simulink library "GFL_Lib"  (R2021a)
settings: Solver=VariableStepAuto  StartTime=0.0  StopTime=10.0  RelTol=1e-3
values from neighbouring files (symbols this model uses):
  Ki_i = Rc_eq*wn_i    [Init_GFL.m]
  Kp_i = Lc_eq/wb*wn_i    [Init_GFL.m]
  Lc_eq = Lc_pu + dLc_pu    [Init_VI_mmc.m]
  Lc_pu = Lt_pu+Larm_pu/2    [Init_VI_mmc.m]
  Lf_pu = Lc_eq    [Init_GFL.m]
  Va0 = sqrt(2)*Vb1*Vvsc0*sin(Theta_vsc0*pi/180)    [Init_LF_LCL_old.m]
  Vb0 = sqrt(2)*Vb1*Vvsc0*sin(Theta_vsc0*pi/180-2*pi/3)    [Init_LF_LCL_old.m]
  Vc0 = sqrt(2)*Vb1*Vvsc0*sin(Theta_vsc0*pi/180+2*pi/3)    [Init_LF_LCL_old.m]
  Vm0_d = Vvsc0 * cos(Theta_vsc0*pi/180-Theta_m0*pi/180)    [Init_LF_LCL_old.m]
  Vm0_q = Vvsc0 * sin(Theta_vsc0*pi/180-Theta_m0*pi/180)    [Init_LF_LCL_old.m]
  Vvsc0 = abs(Vm)    [Init_LF_LCL_old.m]
undefined symbols (not defined in the file or in its folder): Carm, Diff_CC_ki, Diff_CC_kp, fb, Ib2, Idcb, Ki_Wdiff_pu, Ki_Wtot_pu, Kp_Rvi_pu, Kp_Wdiff_pu, Kp_Wtot_pu, Lb, Sb, Solver_Time_Step, Time_Step, Vb1, Vb2, Vdcb, Vm0, VSC01_id0, wb, Zb
libraries: Control_Lib x57, spsVoltageMeasurementLib x17, spsSeriesRLCBranchLib x14, spsThreePhaseSourceLib x12, spsThreePhaseBreakerLib x10, spsThreePhaseVIMeasurementLib x9, spsThreePhaseTransformerTwoWindingsLib x7, spsCurrentMeasurementLib x7, powerlib x7, spsControlledCurrentSourceLib x6, spsControlledVoltageSourceLib x6, slpidlib x6
(part 4 of 6)

== system GFL_Lib/Mean Model 2-Level L-filter_sav/Mean_Model ==
  Uref : Inport
  Constant : Constant
  Memory : Memory
  NOT1 : Logic  Operator=NOT  IconShape=distinctive  AllPortsSameDT=off  OutDataTypeStr=boolean
  Terminator : Terminator
  Three-Phase Breaker1 : spsThreePhaseBreakerLib/Three-Phase Breaker  InitialState=closed  SwitchA=on  SwitchB=on  SwitchC=on  SwitchTimes="[4/60  10/60]"  External=on  BreakerResistance=0.001  SnubberResistance=1e6  SnubberCapacitance=inf  Measurements=None
  Three-Phase Breaker2 : spsThreePhaseBreakerLib/Three-Phase Breaker  InitialState=open  SwitchA=on  SwitchB=on  SwitchC=on  SwitchTimes="[4/60  10/60]"  External=on  BreakerResistance=0.001  SnubberResistance=1e6  SnubberCapacitance=inf  Measurements=None
  Three-Phase Source : spsThreePhaseSourceLib/Three-Phase Source  InternalConnection=Yg  VoltagePhases=off  Voltage=Vvsc0*Un1  PhaseAngle=Theta_vsc0  Voltage_phases=[25e3 25e3 25e3]/sqrt(3)  PhaseAngles_phases=[0 -120 +120]  Frequency=fb  NonIdealSource=off  SpecifyImpedance=off  Resistance=0  Inductance=0  ShortCircuitLevel=100e6  BaseVoltage=VSC01_Un1  XRratio=7  BusType=swing  Pref=0.3  Qref=0  Prefabc=[10e3, 10e3, 10e3]  Qrefabc=[0, 0, 0]  Qmin=-Inf  Qmax=Inf
  Universal Bridge : spsUniversalBridgeLib/Universal Bridge  Arms=3  SnubberResistance=1e5  SnubberCapacitance=inf  Device=Average-model based VSC  Ron=1e-3  Lon=0  ForwardVoltages="[  0  0  ]"  ForwardVoltage=0  GTOparameters=[ 10e-6 , 20e-6 ]  IGBTparameters=[ 1e-6 , 2e-6 ]  Measurements=None  Measurements_2=None  converterType=Rectifier
  Vdc : spsVoltageMeasurementLib/Voltage Measurement  PhasorSimulation=off  OutputType=Complex  PSBequivalent=0
  mp3 : Gain  Gain=2/Udcn
  PhA : PMIOPort  Side=Right
  PhB : PMIOPort  Port=2  Side=Right
  PhC : PMIOPort  Port=3  Side=Right
  Vdc+ : PMIOPort  Port=4  Side=Left
  Vdc- : PMIOPort  Port=5  Side=Left
  wires:
  NOT1/1 -> Three-Phase Breaker1/1
  Memory/1 -> NOT1/1, Three-Phase Breaker2/1
  mp3/1 -> Universal Bridge/1
  Uref/1 -> mp3/1
  Vdc/1 -> Terminator/1
  Constant/1 -> Memory/1
  connections:
  Three-Phase Breaker2/LConn1 -- Three-Phase Breaker1/LConn1 -- PhA/RConn1
  Three-Phase Breaker2/LConn2 -- Three-Phase Breaker1/LConn2 -- PhB/RConn1
  Three-Phase Breaker2/LConn3 -- Three-Phase Breaker1/LConn3 -- PhC/RConn1
  Three-Phase Breaker2/RConn1 -- Universal Bridge/LConn1
  Three-Phase Breaker2/RConn2 -- Universal Bridge/LConn2
  Three-Phase Breaker2/RConn3 -- Universal Bridge/LConn3
  Three-Phase Source/RConn1 -- Three-Phase Breaker1/RConn1
  Three-Phase Source/RConn2 -- Three-Phase Breaker1/RConn2
  Three-Phase Source/RConn3 -- Three-Phase Breaker1/RConn3
  Vdc/LConn1 -- Universal Bridge/RConn1 -- Vdc+/RConn1
  Vdc/LConn2 -- Universal Bridge/RConn2 -- Vdc-/RConn1

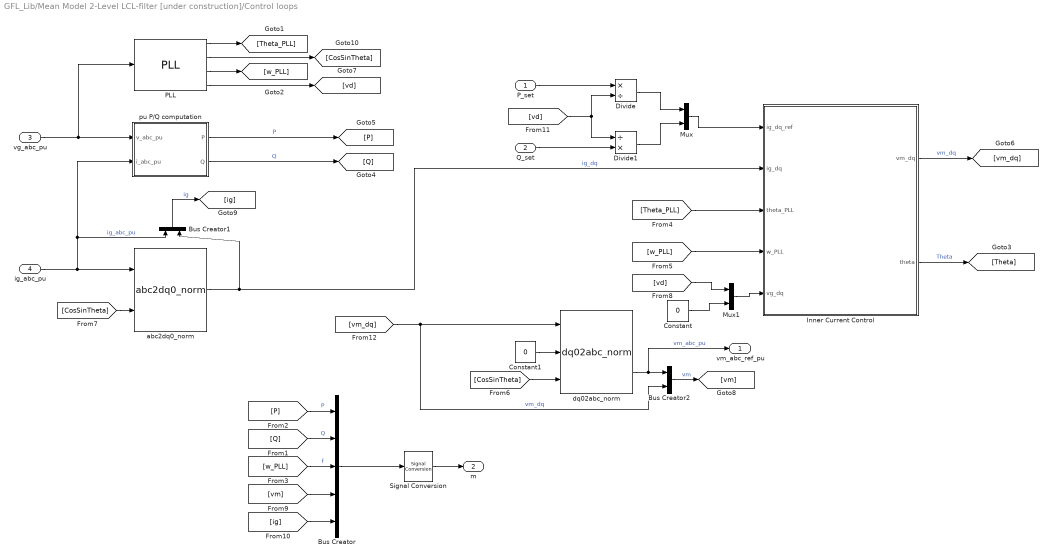
== system GFL_Lib/Mean Model 2-Level LCL-filter [under construction]/Control loops ==
  P_set : Inport
  Q_set : Inport  Port=2
  vg_abc_pu : Inport  Port=3
  ig_abc_pu : Inport  Port=4
  " pu P/Q computation" : Subsystem  DialogController=POWERSYS.PowerSysDialog
  Bus Creator : BusCreator  Inputs=5
  Bus Creator1 : BusCreator  Inputs=2
  Bus Creator2 : BusCreator  Inputs=2
  Constant : Constant  Value=0
  Constant1 : Constant  Value=0
  Divide : Product  Inputs=*/
  Divide1 : Product  Inputs=/*
  Inner Current Control : Subsystem
  Mux : Mux  Inputs=2
  Mux1 : Mux  Inputs=2
  PLL : Control_Lib/PLL  fb=fb  Tr_PLL=Tr_PLL*1000  Theta0=Theta0
      settings: SourceProductName=VSC4SPS
  Signal Conversion : SignalConversion  OverrideOpt=off
  abc2dq0_norm : Control_Lib/abc2dq0_norm  referenceAxisMode=Reference axis at 90 degrees behind phase_a  baseUpdateGain=1/sqrt(3)
      settings: SourceProductName=VSC4SPS
  dq02abc_norm : Control_Lib/dq02abc_norm  referenceAxisMode=Reference axis at 90 degrees behind phase_a  baseUpdateGain=sqrt(3)
      settings: SourceProductName=VSC4SPS
  vm_abc_ref_pu : Outport  VectorParamsAs1DForOutWhenUnconnected=off
  m : Outport  Port=2  VectorParamsAs1DForOutWhenUnconnected=off
  wires:
  PLL/3 -> [w_PLL]
  PLL/1 -> [Theta_PLL]
  [ig] -> Bus Creator/5
  Bus Creator1/1 -> [ig]  "ig"
  Bus Creator/1 -> Signal Conversion/1
  [vm] -> Bus Creator/4
  Bus Creator2/1 -> [vm]  "vm"
  [CosSinTheta] -> abc2dq0_norm/2
  [CosSinTheta] -> dq02abc_norm/3
  Inner Current Control/2(theta) -> [Theta]  "Theta"
  abc2dq0_norm/2 -> Bus Creator1/2, Inner Current Control/2(ig_dq)  "ig_dq"
  ig_abc_pu/1 -> " pu P/Q computation"/2(i_abc_pu), Bus Creator1/1, abc2dq0_norm/1  "ig_abc_pu"
  " pu P/Q computation"/1(P) -> [P]  "P"
  vg_abc_pu/1 -> " pu P/Q computation"/1(v_abc_pu), PLL/1
  Inner Current Control/1(vm_dq) -> [vm_dq]  "vm_dq"
  [w_PLL] -> Inner Current Control/4(w_PLL)
  P_set/1 -> Divide/1
  [Theta_PLL] -> Inner Current Control/3(theta_PLL)
  [vm_dq] -> dq02abc_norm/1, Bus Creator2/2  "vm_dq"
  " pu P/Q computation"/2(Q) -> [Q]  "Q"
  Q_set/1 -> Divide1/2
  dq02abc_norm/2 -> vm_abc_ref_pu/1, Bus Creator2/1  "vm_abc_pu"
  [w_PLL] -> Bus Creator/3  "f"
  [Q] -> Bus Creator/2  "Q"
  [P] -> Bus Creator/1  "P"
  Signal Conversion/1 -> m/1
  PLL/4 -> [vd]
  [vd] -> Divide/2, Divide1/1
  Divide/1 -> Mux/1
  Divide1/1 -> Mux/2
  Mux/1 -> Inner Current Control/1(ig_dq_ref)
  [vd] -> Mux1/1
  Mux1/1 -> Inner Current Control/5(vg_dq)
  Constant/1 -> Mux1/2
  PLL/2 -> [CosSinTheta]
  Constant1/1 -> dq02abc_norm/2

== system GFL_Lib/Mean Model 2-Level LCL-filter [under construction]/Mean_model ==
  Uref : Inport
  Constant : Constant
  Memory : Memory
  NOT1 : Logic  Operator=NOT  IconShape=distinctive  AllPortsSameDT=off  OutDataTypeStr=boolean
  Terminator : Terminator
  Three-Phase Breaker1 : powerlib/Elements/Three-Phase Breaker  InitialState=closed  SwitchA=on  SwitchB=on  SwitchC=on  SwitchTimes="[4/60  10/60]"  External=on  BreakerResistance=0.001  SnubberResistance=1e6  SnubberCapacitance=inf  Measurements=None
  Three-Phase Breaker2 : powerlib/Elements/Three-Phase Breaker  InitialState=open  SwitchA=on  SwitchB=on  SwitchC=on  SwitchTimes="[4/60  10/60]"  External=on  BreakerResistance=0.001  SnubberResistance=1e6  SnubberCapacitance=inf  Measurements=None
  Three-Phase Source : powerlib/Electrical Sources/Three-Phase Source  InternalConnection=Yg  VoltagePhases=off  Voltage=Vvsc0*Un1  PhaseAngle=Theta_vsc0  Voltage_phases=[25e3 25e3 25e3]/sqrt(3)  PhaseAngles_phases=[0 -120 +120]  Frequency=fb  NonIdealSource=off  SpecifyImpedance=off  Resistance=0  Inductance=0  ShortCircuitLevel=100e6  BaseVoltage=VSC01_Un1  XRratio=7  BusType=swing  Pref=0.3  Qref=0  Prefabc=[10e3, 10e3, 10e3]  Qrefabc=[0, 0, 0]  Qmin=-Inf  Qmax=Inf
  Universal Bridge : powerlib/Power Electronics/Universal Bridge  Arms=3  SnubberResistance=1e5  SnubberCapacitance=inf  Device=Average-model based VSC  Ron=1e-3  Lon=0  ForwardVoltages="[  0  0  ]"  ForwardVoltage=0  GTOparameters=[ 10e-6 , 20e-6 ]  IGBTparameters=[ 1e-6 , 2e-6 ]  Measurements=None  Measurements_2=None  converterType=Rectifier
  Vdc : powerlib/Measurements/Voltage Measurement  PhasorSimulation=off  OutputType=Complex  PSBequivalent=0
  mp3 : Gain  Gain=2/Udcn
  PhA : PMIOPort  Side=Right
  PhB : PMIOPort  Port=2  Side=Right
  PhC : PMIOPort  Port=3  Side=Right
  Vdc+ : PMIOPort  Port=4  Side=Left
  Vdc- : PMIOPort  Port=5  Side=Left
  wires:
  NOT1/1 -> Three-Phase Breaker1/1
  Memory/1 -> NOT1/1, Three-Phase Breaker2/1
  mp3/1 -> Universal Bridge/1
  Uref/1 -> mp3/1
  Vdc/1 -> Terminator/1
  Constant/1 -> Memory/1
  connections:
  Three-Phase Breaker2/LConn1 -- Three-Phase Breaker1/LConn1 -- PhA/RConn1
  Three-Phase Breaker2/LConn2 -- Three-Phase Breaker1/LConn2 -- PhB/RConn1
  Three-Phase Breaker2/LConn3 -- Three-Phase Breaker1/LConn3 -- PhC/RConn1
  Three-Phase Breaker2/RConn1 -- Universal Bridge/LConn1
  Three-Phase Breaker2/RConn2 -- Universal Bridge/LConn2
  Three-Phase Breaker2/RConn3 -- Universal Bridge/LConn3
  Three-Phase Source/RConn1 -- Three-Phase Breaker1/RConn1
  Three-Phase Source/RConn2 -- Three-Phase Breaker1/RConn2
  Three-Phase Source/RConn3 -- Three-Phase Breaker1/RConn3
  Vdc/LConn1 -- Universal Bridge/RConn1 -- Vdc+/RConn1
  Vdc/LConn2 -- Universal Bridge/RConn2 -- Vdc-/RConn1

== system GFL_Lib/GFL IDEAL VSC/Control loops/ pu P//Q computation ==
  v_abc_pu : Inport  PortDimensions=3
  i_abc_pu : Inport  Port=2  PortDimensions=3
  Demux : Demux  Outputs=3
      settings: DisplayOption=none
  Mux : Mux  Inputs=3
  Product1 : Product  InputSameDT=on  SaturateOnIntegerOverflow=on  OutDataTypeStr=Inherit: Same as first input
  Product3 : Product  InputSameDT=on  SaturateOnIntegerOverflow=on  OutDataTypeStr=Inherit: Same as first input
  Sum : Sum  Inputs=+-  InputSameDT=on  SaturateOnIntegerOverflow=on  OutDataTypeStr=Inherit: Same as first input
  Sum1 : Sum  Inputs=1  InputSameDT=on  SaturateOnIntegerOverflow=on  OutDataTypeStr=Inherit: Same as first input
  Sum4 : Sum  Inputs=1  InputSameDT=on  SaturateOnIntegerOverflow=on  OutDataTypeStr=Inherit: Same as first input
  Sum5 : Sum  Inputs=+-  InputSameDT=on  SaturateOnIntegerOverflow=on  OutDataTypeStr=Inherit: Same as first input
  Sum6 : Sum  Inputs=+-  InputSameDT=on  SaturateOnIntegerOverflow=on  OutDataTypeStr=Inherit: Same as first input
  pu->V : Gain  Gain=1/sqrt(3)  SaturateOnIntegerOverflow=on  OutDataTypeStr=Inherit: Same as input  ParamDataTypeStr=Inherit: Same as input
  pu->V1 : Gain  Gain=1/3  SaturateOnIntegerOverflow=on  OutDataTypeStr=Inherit: Same as input  ParamDataTypeStr=Inherit: Same as input
  pu->V2 : Gain  Gain=1/3  SaturateOnIntegerOverflow=on  OutDataTypeStr=Inherit: Same as input  ParamDataTypeStr=Inherit: Same as input
  P : Outport  VectorParamsAs1DForOutWhenUnconnected=off
  Q : Outport  Port=2  VectorParamsAs1DForOutWhenUnconnected=off
  wires:
  pu->V2/1 -> Q/1
  pu->V1/1 -> P/1
  Sum1/1 -> pu->V/1
  Product3/1 -> Sum1/1
  Product1/1 -> Sum4/1
  v_abc_pu/1 -> Product1/1, Demux/1
  i_abc_pu/1 -> Product1/2, Product3/2
  Sum4/1 -> pu->V1/1
  Demux/1 -> Sum/1, Sum6/2
  Demux/2 -> Sum/2, Sum5/1
  Demux/3 -> Sum5/2, Sum6/1
  Sum/1 -> Mux/3
  Sum5/1 -> Mux/1
  Sum6/1 -> Mux/2
  Mux/1 -> Product3/1
  pu->V/1 -> pu->V2/1  "Q"

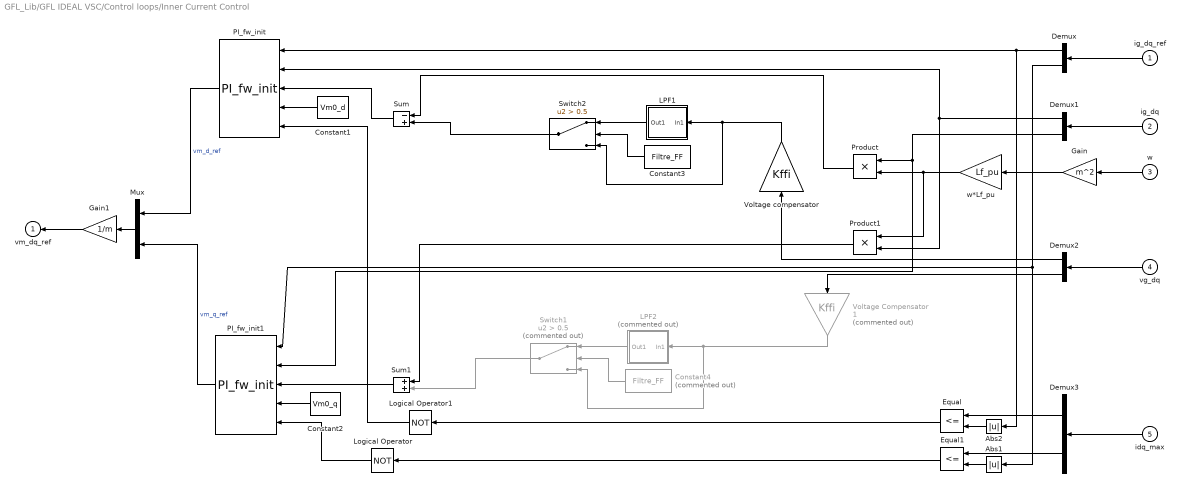
== system GFL_Lib/GFL IDEAL VSC/Control loops/Inner Current Control ==
  ig_dq_ref : Inport
  ig_dq : Inport  Port=2
  w : Inport  Port=3
  vg_dq : Inport  Port=4
  idq_max : Inport  Port=5
  Abs1 : Abs
  Abs2 : Abs
  Constant1 : Constant  Value=Vm0_d
  Constant2 : Constant  Value=Vm0_q
  Constant3 : Constant  Value=Filtre_FF
  Constant4 : Constant  Commented=on  Value=Filtre_FF
  Demux{,1..3} (4 alike) : Demux  Outputs=2
  Equal : RelationalOperator  Operator=<=  OutDataTypeStr=boolean  RndMeth=Simplest
  Equal1 : RelationalOperator  Operator=<=  OutDataTypeStr=boolean  RndMeth=Simplest
  Gain : Gain  Gain=m^2
  Gain1 : Gain  Gain=1/m
  LPF1 : Subsystem
  LPF2 : Subsystem  Commented=on
  Logical Operator : Logic  Operator=NOT  AllPortsSameDT=off  OutDataTypeStr=boolean
  Logical Operator1 : Logic  Operator=NOT  AllPortsSameDT=off  OutDataTypeStr=boolean
  Mux : Mux  Inputs=[1 1]
  PI_fw_init : Control_Lib/PI_fw_init  Kp=Kp_i  Ki=Ki_i
      settings: SourceProductName=VSC4SPS
  PI_fw_init1 : Control_Lib/PI_fw_init  Kp=Kp_i  Ki=Ki_i
      settings: SourceProductName=VSC4SPS
  Product : Product  RndMeth=Zero
  Product1 : Product  RndMeth=Zero
  Sum : Sum  Inputs=-+
  Sum1 : Sum
  Switch1 : Switch  Commented=on  Criteria=u2 > Threshold  Threshold=0.5
  Switch2 : Switch  Criteria=u2 > Threshold  Threshold=0.5
  Voltage Compensator 1 : Gain  Commented=on  Gain=Kffi
  Voltage compensator : Gain  Gain=Kffi
  w*Lf_pu : Gain  Gain=Lf_pu
  vm_dq_ref : Outport  InitialOutput=0  VectorParamsAs1DForOutWhenUnconnected=off
  wires:
  Switch1/1 -> Sum1/2
  Constant4/1 -> Switch1/2
  Voltage Compensator 1/1 -> LPF2/1(In1), Switch1/3
  LPF2/1(Out1) -> Switch1/1
  Constant3/1 -> Switch2/2
  LPF1/1(Out1) -> Switch2/1
  Gain1/1 -> vm_dq_ref/1
  Gain/1 -> w*Lf_pu/1
  Equal1/1 -> Logical Operator/1
  Equal/1 -> Logical Operator1/1
  Abs1/1 -> Equal1/2
  Abs2/1 -> Equal/2
  Demux3/2 -> Equal1/1
  Demux3/1 -> Equal/1
  idq_max/1 -> Demux3/1
  Demux2/2 -> Voltage Compensator 1/1
  Demux2/1 -> Voltage compensator/1
  Constant2/1 -> PI_fw_init1/4
  Constant1/1 -> PI_fw_init/4
  Product/1 -> Sum/1
  vg_dq/1 -> Demux2/1
  ig_dq/1 -> Demux1/1
  ig_dq_ref/1 -> Demux/1
  Demux/1 -> Abs2/1, PI_fw_init/1
  Demux1/1 -> Product1/2, PI_fw_init/2
  w*Lf_pu/1 -> Product1/1, Product/2
  Demux1/2 -> Product/1, PI_fw_init1/2
  Mux/1 -> Gain1/1
  Demux/2 -> PI_fw_init1/1, Abs1/1
  Product1/1 -> Sum1/1
  PI_fw_init/1 -> Mux/1  "vm_d_ref"
  PI_fw_init1/1 -> Mux/2  "vm_q_ref"
  w/1 -> Gain/1
  Voltage compensator/1 -> LPF1/1(In1), Switch2/3
  Sum/1 -> PI_fw_init/3
  Sum1/1 -> PI_fw_init1/3
  Switch2/1 -> Sum/2
  Logical Operator/1 -> PI_fw_init1/5
  Logical Operator1/1 -> PI_fw_init/5

== system GFL_Lib/GFL IDEAL VSC/Control loops/LPF ==
  In1 : Inport
  Add : Sum  Inputs=+-
  Gain : Gain  Gain=w_LPF
  Integrator : Integrator  InitialConditionSource=external  InitialCondition=P0
  Out1 : Outport
  wires:
  Add/1 -> Gain/1
  Gain/1 -> Integrator/1
  Integrator/1 -> Out1/1, Add/2
  In1/1 -> Integrator/2, Add/1

== system GFL_Lib/GFL IDEAL VSC/Control loops/LPF1 ==
  In1 : Inport
  Add : Sum  Inputs=+-
  Gain : Gain  Gain=w_LPF
  Integrator : Integrator  InitialConditionSource=external  InitialCondition=V0
  Ref : Outport
  wires:
  Add/1 -> Gain/1
  Gain/1 -> Integrator/1
  Integrator/1 -> Ref/1, Add/2
  In1/1 -> Integrator/2, Add/1

== system GFL_Lib/GFL IDEAL VSC/Control loops/LPF2 ==
  In1 : Inport
  Add : Sum  Inputs=+-
  Gain : Gain  Gain=w_LPF
  Integrator : Integrator  InitialConditionSource=external  InitialCondition=Q0
  Out1 : Outport
  wires:
  Add/1 -> Gain/1
  Gain/1 -> Integrator/1
  Integrator/1 -> Out1/1, Add/2
  In1/1 -> Integrator/2, Add/1

== system GFL_Lib/GFL IDEAL VSC/Control loops/LPF3 ==
  In1 : Inport
  Add : Sum  Inputs=+-
  Gain : Gain  Gain=2*pi*50
  Integrator : Integrator  InitialConditionSource=external  InitialCondition=V0
  Out1 : Outport
  wires:
  Add/1 -> Gain/1
  Gain/1 -> Integrator/1
  Integrator/1 -> Out1/1, Add/2
  In1/1 -> Integrator/2, Add/1

== system GFL_Lib/GFL IDEAL VSC/Control loops/RMS derivation ==
  dq : Inport
  Demux : Demux  Outputs=2
  Sqrt : Sqrt  SaturateOnIntegerOverflow=on
  Square : Math  Operator=square  SaturateOnIntegerOverflow=on
  Square1 : Math  Operator=square  SaturateOnIntegerOverflow=on
  Sum : Sum
  rms : Outport
  wires:
  Square1/1 -> Sum/2
  Sum/1 -> Sqrt/1
  Sqrt/1 -> rms/1
  Demux/1 -> Square/1
  Square/1 -> Sum/1
  Demux/2 -> Square1/1
  dq/1 -> Demux/1

== system GFL_Lib/GFL IDEAL VSC/Control loops/RMS derivation1 ==
  dq : Inport
  Demux : Demux  Outputs=2
  Sqrt : Sqrt  SaturateOnIntegerOverflow=on
  Square : Math  Operator=square  SaturateOnIntegerOverflow=on
  Square1 : Math  Operator=square  SaturateOnIntegerOverflow=on
  Sum : Sum
  rms : Outport
  wires:
  dq/1 -> Demux/1
  Demux/2 -> Square1/1
  Square/1 -> Sum/1
  Demux/1 -> Square/1
  Sqrt/1 -> rms/1
  Sum/1 -> Sqrt/1
  Square1/1 -> Sum/2

== system GFL_Lib/GFL IDEAL VSC/Control loops/RMS derivation2 ==
  dq : Inport
  Demux : Demux  Outputs=2
  Sqrt : Sqrt  SaturateOnIntegerOverflow=on
  Square : Math  Operator=square  SaturateOnIntegerOverflow=on
  Square1 : Math  Operator=square  SaturateOnIntegerOverflow=on
  Sum : Sum
  rms : Outport
  wires:
  dq/1 -> Demux/1
  Demux/2 -> Square1/1
  Square/1 -> Sum/1
  Demux/1 -> Square/1
  Sqrt/1 -> rms/1
  Sum/1 -> Sqrt/1
  Square1/1 -> Sum/2

== system GFL_Lib/GFL IDEAL VSC/Control loops/norm1 ==
  In1 : Inport
  Add : Sum
  Demux : Demux  Outputs=2
  Sqrt : Sqrt  SaturateOnIntegerOverflow=on
  Square : Math  Operator=square  SaturateOnIntegerOverflow=on
  Square1 : Math  Operator=square  SaturateOnIntegerOverflow=on
  Out1 : Outport
  wires:
  Sqrt/1 -> Out1/1
  Add/1 -> Sqrt/1
  Demux/2 -> Square1/1
  Demux/1 -> Square/1
  Square/1 -> Add/1
  Square1/1 -> Add/2
  In1/1 -> Demux/1

== system GFL_Lib/GFL IDEAL VSC/Control loops/norm2 ==
  In1 : Inport
  Add : Sum
  Demux : Demux  Outputs=2
  Sqrt : Sqrt  SaturateOnIntegerOverflow=on
  Square : Math  Operator=square  SaturateOnIntegerOverflow=on
  Square1 : Math  Operator=square  SaturateOnIntegerOverflow=on
  Out1 : Outport
  wires:
  Sqrt/1 -> Out1/1
  Add/1 -> Sqrt/1
  Demux/2 -> Square1/1
  Demux/1 -> Square/1
  Square/1 -> Add/1
  Square1/1 -> Add/2
  In1/1 -> Demux/1

== system GFL_Lib/GFL MMC/Control loops/ pu P//Q computation ==
  v_abc_pu : Inport  PortDimensions=3
  i_abc_pu : Inport  Port=2  PortDimensions=3
  Demux : Demux  Outputs=3
      settings: DisplayOption=none
  Mux : Mux  Inputs=3
  Product1 : Product  InputSameDT=on  SaturateOnIntegerOverflow=on  OutDataTypeStr=Inherit: Same as first input
  Product3 : Product  InputSameDT=on  SaturateOnIntegerOverflow=on  OutDataTypeStr=Inherit: Same as first input
  Sum : Sum  Inputs=+-  InputSameDT=on  SaturateOnIntegerOverflow=on  OutDataTypeStr=Inherit: Same as first input
  Sum1 : Sum  Inputs=1  InputSameDT=on  SaturateOnIntegerOverflow=on  OutDataTypeStr=Inherit: Same as first input
  Sum4 : Sum  Inputs=1  InputSameDT=on  SaturateOnIntegerOverflow=on  OutDataTypeStr=Inherit: Same as first input
  Sum5 : Sum  Inputs=+-  InputSameDT=on  SaturateOnIntegerOverflow=on  OutDataTypeStr=Inherit: Same as first input
  Sum6 : Sum  Inputs=+-  InputSameDT=on  SaturateOnIntegerOverflow=on  OutDataTypeStr=Inherit: Same as first input
  pu->V : Gain  Gain=1/sqrt(3)  SaturateOnIntegerOverflow=on  OutDataTypeStr=Inherit: Same as input  ParamDataTypeStr=Inherit: Same as input
  pu->V1 : Gain  Gain=1/3  SaturateOnIntegerOverflow=on  OutDataTypeStr=Inherit: Same as input  ParamDataTypeStr=Inherit: Same as input
  pu->V2 : Gain  Gain=1/3  SaturateOnIntegerOverflow=on  OutDataTypeStr=Inherit: Same as input  ParamDataTypeStr=Inherit: Same as input
  P : Outport  VectorParamsAs1DForOutWhenUnconnected=off
  Q : Outport  Port=2  VectorParamsAs1DForOutWhenUnconnected=off
  wires:
  pu->V2/1 -> Q/1
  pu->V1/1 -> P/1
  Sum1/1 -> pu->V/1
  Product3/1 -> Sum1/1
  Product1/1 -> Sum4/1
  v_abc_pu/1 -> Product1/1, Demux/1
  i_abc_pu/1 -> Product1/2, Product3/2
  Sum4/1 -> pu->V1/1
  Demux/1 -> Sum/1, Sum6/2
  Demux/2 -> Sum/2, Sum5/1
  Demux/3 -> Sum5/2, Sum6/1
  Sum/1 -> Mux/3
  Sum5/1 -> Mux/1
  Sum6/1 -> Mux/2
  Mux/1 -> Product3/1
  pu->V/1 -> pu->V2/1  "Q"

== system GFL_Lib/GFL MMC/Control loops/Inner Current Control ==
  ig_dq_ref : Inport
  ig_dq : Inport  Port=2
  w : Inport  Port=3
  vg_dq : Inport  Port=4
  idq_max : Inport  Port=5
  Abs1 : Abs
  Abs2 : Abs
  Constant1 : Constant  Value=Vm0_d
  Constant2 : Constant  Value=Vm0_q
  Constant3 : Constant  Value=Filtre_FF
  Constant4 : Constant  Commented=on  Value=Filtre_FF
  Demux{,1..3} (4 alike) : Demux  Outputs=2
  Equal : RelationalOperator  Operator=<=  OutDataTypeStr=boolean  RndMeth=Simplest
  Equal1 : RelationalOperator  Operator=<=  OutDataTypeStr=boolean  RndMeth=Simplest
  Gain : Gain  Gain=m^2
  Gain1 : Gain  Gain=1/m
  LPF1 : Subsystem
  LPF2 : Subsystem  Commented=on
  Logical Operator : Logic  Operator=NOT  AllPortsSameDT=off  OutDataTypeStr=boolean
  Logical Operator1 : Logic  Operator=NOT  AllPortsSameDT=off  OutDataTypeStr=boolean
  Mux : Mux  Inputs=[1 1]
  PI_fw_init : Control_Lib/PI_fw_init  Kp=Kp_i  Ki=Ki_i
      settings: SourceProductName=VSC4SPS
  PI_fw_init1 : Control_Lib/PI_fw_init  Kp=Kp_i  Ki=Ki_i
      settings: SourceProductName=VSC4SPS
  Product : Product  RndMeth=Zero
  Product1 : Product  RndMeth=Zero
  Sum : Sum  Inputs=-+
  Sum1 : Sum
  Switch1 : Switch  Commented=on  Criteria=u2 > Threshold  Threshold=0.5
  Switch2 : Switch  Criteria=u2 > Threshold  Threshold=0.5
  Voltage Compensator 1 : Gain  Commented=on  Gain=Kffi
  Voltage compensator : Gain  Gain=Kffi
  w*Lf_pu : Gain  Gain=Lf_pu
  vm_dq_ref : Outport  InitialOutput=0  VectorParamsAs1DForOutWhenUnconnected=off
  wires:
  Switch1/1 -> Sum1/2
  Constant4/1 -> Switch1/2
  Voltage Compensator 1/1 -> LPF2/1(In1), Switch1/3
  LPF2/1(Out1) -> Switch1/1
  Constant3/1 -> Switch2/2
  LPF1/1(Out1) -> Switch2/1
  Gain1/1 -> vm_dq_ref/1
  Gain/1 -> w*Lf_pu/1
  Equal1/1 -> Logical Operator/1
  Equal/1 -> Logical Operator1/1
  Abs1/1 -> Equal1/2
  Abs2/1 -> Equal/2
  Demux3/2 -> Equal1/1
  Demux3/1 -> Equal/1
  idq_max/1 -> Demux3/1
  Demux2/2 -> Voltage Compensator 1/1
  Demux2/1 -> Voltage compensator/1
  Constant2/1 -> PI_fw_init1/4
  Constant1/1 -> PI_fw_init/4
  Product/1 -> Sum/1
  vg_dq/1 -> Demux2/1
  ig_dq/1 -> Demux1/1
  ig_dq_ref/1 -> Demux/1
  Demux/1 -> Abs2/1, PI_fw_init/1
  Demux1/1 -> Product1/2, PI_fw_init/2
  w*Lf_pu/1 -> Product1/1, Product/2
  Demux1/2 -> Product/1, PI_fw_init1/2
  Mux/1 -> Gain1/1
  Demux/2 -> PI_fw_init1/1, Abs1/1
  Product1/1 -> Sum1/1
  PI_fw_init/1 -> Mux/1  "vm_d_ref"
  PI_fw_init1/1 -> Mux/2  "vm_q_ref"
  w/1 -> Gain/1
  Voltage compensator/1 -> LPF1/1(In1), Switch2/3
  Sum/1 -> PI_fw_init/3
  Sum1/1 -> PI_fw_init1/3
  Switch2/1 -> Sum/2
  Logical Operator/1 -> PI_fw_init1/5
  Logical Operator1/1 -> PI_fw_init/5

== system GFL_Lib/GFL MMC/Control loops/LPF ==
  In1 : Inport
  Add : Sum  Inputs=+-
  Gain : Gain  Gain=w_LPF
  Integrator : Integrator  InitialConditionSource=external  InitialCondition=P0
  Out1 : Outport
  wires:
  Add/1 -> Gain/1
  Gain/1 -> Integrator/1
  Integrator/1 -> Out1/1, Add/2
  In1/1 -> Integrator/2, Add/1

== system GFL_Lib/GFL MMC/Control loops/LPF1 ==
  In1 : Inport
  Add : Sum  Inputs=+-
  Gain : Gain  Gain=w_LPF
  Integrator : Integrator  InitialConditionSource=external  InitialCondition=V0
  Out1 : Outport
  wires:
  Add/1 -> Gain/1
  Gain/1 -> Integrator/1
  Integrator/1 -> Out1/1, Add/2
  In1/1 -> Integrator/2, Add/1

== system GFL_Lib/GFL MMC/Control loops/LPF2 ==
  In1 : Inport
  Add : Sum  Inputs=+-
  Gain : Gain  Gain=w_LPF
  Integrator : Integrator  InitialConditionSource=external  InitialCondition=Q0
  Out1 : Outport
  wires:
  Add/1 -> Gain/1
  Gain/1 -> Integrator/1
  Integrator/1 -> Out1/1, Add/2
  In1/1 -> Integrator/2, Add/1

== system GFL_Lib/GFL MMC/Control loops/LPF3 ==
  In1 : Inport
  Add : Sum  Inputs=+-
  Gain : Gain  Gain=2*pi*50
  Integrator : Integrator  InitialConditionSource=external  InitialCondition=V0
  Out1 : Outport
  wires:
  Add/1 -> Gain/1
  Gain/1 -> Integrator/1
  Integrator/1 -> Out1/1, Add/2
  In1/1 -> Integrator/2, Add/1

== system GFL_Lib/GFL MMC/Control loops/RMS derivation ==
  dq : Inport
  Demux : Demux  Outputs=2
  Sqrt : Sqrt  SaturateOnIntegerOverflow=on
  Square : Math  Operator=square  SaturateOnIntegerOverflow=on
  Square1 : Math  Operator=square  SaturateOnIntegerOverflow=on
  Sum : Sum
  rms : Outport
  wires:
  Square1/1 -> Sum/2
  Sum/1 -> Sqrt/1
  Sqrt/1 -> rms/1
  Demux/1 -> Square/1
  Square/1 -> Sum/1
  Demux/2 -> Square1/1
  dq/1 -> Demux/1

== system GFL_Lib/GFL MMC/Control loops/RMS derivation1 ==
  dq : Inport
  Demux : Demux  Outputs=2
  Sqrt : Sqrt  SaturateOnIntegerOverflow=on
  Square : Math  Operator=square  SaturateOnIntegerOverflow=on
  Square1 : Math  Operator=square  SaturateOnIntegerOverflow=on
  Sum : Sum
  rms : Outport
  wires:
  dq/1 -> Demux/1
  Demux/2 -> Square1/1
  Square/1 -> Sum/1
  Demux/1 -> Square/1
  Sqrt/1 -> rms/1
  Sum/1 -> Sqrt/1
  Square1/1 -> Sum/2

== system GFL_Lib/GFL MMC/Control loops/RMS derivation2 ==
  dq : Inport
  Demux : Demux  Outputs=2
  Sqrt : Sqrt  SaturateOnIntegerOverflow=on
  Square : Math  Operator=square  SaturateOnIntegerOverflow=on
  Square1 : Math  Operator=square  SaturateOnIntegerOverflow=on
  Sum : Sum
  rms : Outport
  wires:
  dq/1 -> Demux/1
  Demux/2 -> Square1/1
  Square/1 -> Sum/1
  Demux/1 -> Square/1
  Sqrt/1 -> rms/1
  Sum/1 -> Sqrt/1
  Square1/1 -> Sum/2

== system GFL_Lib/GFL MMC/Control loops/norm1 ==
  In1 : Inport
  Add : Sum
  Demux : Demux  Outputs=2
  Sqrt : Sqrt  SaturateOnIntegerOverflow=on
  Square : Math  Operator=square  SaturateOnIntegerOverflow=on
  Square1 : Math  Operator=square  SaturateOnIntegerOverflow=on
  Out1 : Outport
  wires:
  Sqrt/1 -> Out1/1
  Add/1 -> Sqrt/1
  Demux/2 -> Square1/1
  Demux/1 -> Square/1
  Square/1 -> Add/1
  Square1/1 -> Add/2
  In1/1 -> Demux/1

== system GFL_Lib/GFL MMC/Control loops/norm2 ==
  In1 : Inport
  Add : Sum
  Demux : Demux  Outputs=2
  Sqrt : Sqrt  SaturateOnIntegerOverflow=on
  Square : Math  Operator=square  SaturateOnIntegerOverflow=on
  Square1 : Math  Operator=square  SaturateOnIntegerOverflow=on
  Out1 : Outport
  wires:
  Sqrt/1 -> Out1/1
  Add/1 -> Sqrt/1
  Demux/2 -> Square1/1
  Demux/1 -> Square/1
  Square/1 -> Add/1
  Square1/1 -> Add/2
  In1/1 -> Demux/1

== system GFL_Lib/GFM_VC MMC/Bridge_Model/Decoupling voltage ==
  Vv_ref : Inport
  Vdiff_ref : Inport  Port=2
  Sum7 : Sum  Inputs=+-
  Sum8 : Sum
  Vmu_ref : Outport
  Vml_ref : Outport  Port=2
  wires:
  Sum8/1 -> Vml_ref/1  "Ul"
  Sum7/1 -> Vmu_ref/1
  Vdiff_ref/1 -> Sum8/1, Sum7/1
  Vv_ref/1 -> Sum8/2, Sum7/2

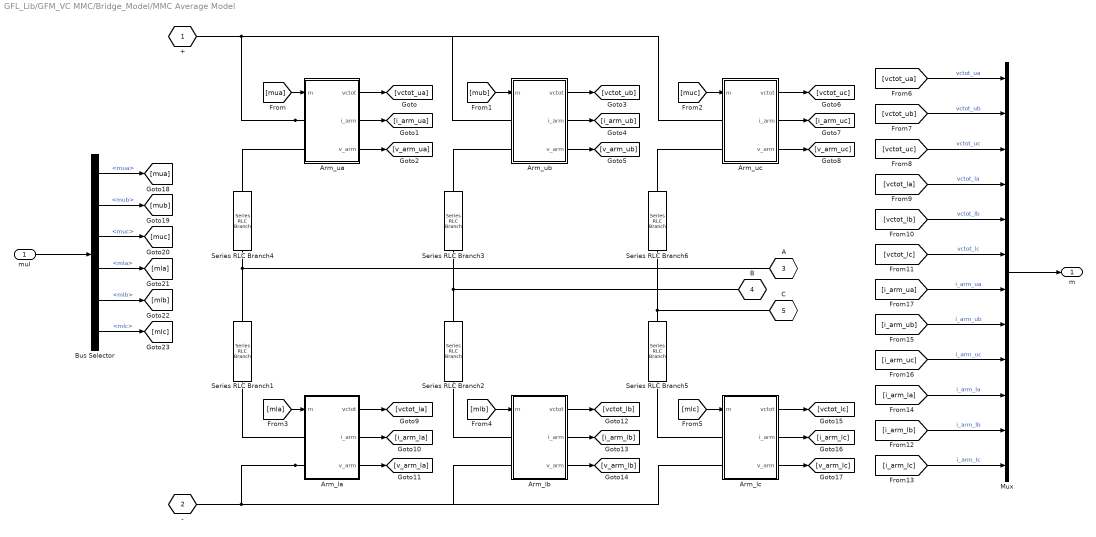
== system GFL_Lib/GFM_VC MMC/Bridge_Model/MMC Average Model ==
  mul : Inport
  Arm_la : Subsystem  mask{C_arm=Carm, Vdc=Udcn}
      mask prompts: C_arm "Arm equivalent Capacitor (F)"; Vdc "Init DC Voltage (V)"
  Arm_lb : Subsystem  mask{C_arm=Carm, Vdc=Udcn}
      mask prompts: C_arm "Arm equivalent Capacitor (F)"; Vdc "Init DC Voltage (V)"
  Arm_lc : Subsystem  mask{C_arm=Carm, Vdc=Udcn}
      mask prompts: C_arm "Arm equivalent Capacitor (F)"; Vdc "Init DC Voltage (V)"
  Arm_ua : Subsystem  mask{C_arm=Carm, Vdc=Udcn}
      mask prompts: C_arm "Arm equivalent Capacitor (F)"; Vdc "Init DC Voltage (V)"
  Arm_ub : Subsystem  mask{C_arm=Carm, Vdc=Udcn}
      mask prompts: C_arm "Arm equivalent Capacitor (F)"; Vdc "Init DC Voltage (V)"
  Arm_uc : Subsystem  mask{C_arm=Carm, Vdc=Udcn}
      mask prompts: C_arm "Arm equivalent Capacitor (F)"; Vdc "Init DC Voltage (V)"
  Bus Selector : BusSelector  OutputSignals=mua,mub,muc,mla,mlb,mlc
  Mux : Mux  Inputs=12
  Series RLC Branch{1..6} (6 alike) : spsSeriesRLCBranchLib/Series RLC Branch  LConnTagsString=__new0  RConnTagsString=__new0  BranchType=RL  Resistance=Rarm_pu*Zb  Inductance=Larm_pu*Lb  SetiL0=off  InitialCurrent=0  Capacitance=1e-6  Setx0=off  InitialVoltage=0  Measurements=None
  + : PMIOPort  Tag=PMCPort  Side=Right
  - : PMIOPort  Tag=PMCPort  Port=2  Side=Right
  A : PMIOPort  Tag=PMCPort  Port=3  Side=Left
  B : PMIOPort  Tag=PMCPort  Port=4  Side=Left
  C : PMIOPort  Tag=PMCPort  Port=5  Side=Left
  m : Outport
  wires:
  [mlb] -> Arm_lb/1(m)
  [mlc] -> Arm_lc/1(m)
  [mla] -> Arm_la/1(m)
  Arm_uc/1(vctot) -> [vctot_uc]
  Arm_lb/3(v_arm) -> [v_arm_lb]
  Arm_ub/3(v_arm) -> [v_arm_ub]
  Arm_ua/1(vctot) -> [vctot_ua]
  Arm_uc/2(i_arm) -> [i_arm_uc]
  Arm_lc/1(vctot) -> [vctot_lc]
  Arm_la/2(i_arm) -> [i_arm_la]
  Arm_la/1(vctot) -> [vctot_la]
  Arm_ub/2(i_arm) -> [i_arm_ub]
  Arm_lc/3(v_arm) -> [v_arm_lc]
  Arm_la/3(v_arm) -> [v_arm_la]
  [mua] -> Arm_ua/1(m)
  Arm_ub/1(vctot) -> [vctot_ub]
  Arm_lb/1(vctot) -> [vctot_lb]
  [mub] -> Arm_ub/1(m)
  Arm_uc/3(v_arm) -> [v_arm_uc]
  Arm_lb/2(i_arm) -> [i_arm_lb]
  Arm_ua/2(i_arm) -> [i_arm_ua]
  Arm_lc/2(i_arm) -> [i_arm_lc]
  [muc] -> Arm_uc/1(m)
  Arm_ua/3(v_arm) -> [v_arm_ua]
  mul/1 -> Bus Selector/1
  Bus Selector/1 -> [mua]  "<mua>"
  Bus Selector/2 -> [mub]  "<mub>"
  Bus Selector/3 -> [muc]  "<muc>"
  Bus Selector/6 -> [mlc]  "<mlc>"
  Bus Selector/5 -> [mlb]  "<mlb>"
  Bus Selector/4 -> [mla]  "<mla>"
  [vctot_lc] -> Mux/6  "vctot_lc"
  [vctot_uc] -> Mux/3  "vctot_uc"
  [i_arm_ua] -> Mux/7  "i_arm_ua"
  [i_arm_ub] -> Mux/8  "i_arm_ub"
  [vctot_lb] -> Mux/5  "vctot_lb"
  [i_arm_la] -> Mux/10  "i_arm_la"
  [vctot_ub] -> Mux/2  "vctot_ub"
  [i_arm_uc] -> Mux/9  "i_arm_uc"
  [vctot_la] -> Mux/4  "vctot_la"
  [i_arm_lb] -> Mux/11  "i_arm_lb"
  [vctot_ua] -> Mux/1  "vctot_ua"
  [i_arm_lc] -> Mux/12  "i_arm_lc"
  Mux/1 -> m/1
  connections:
  Series RLC Branch5/RConn1 -- Arm_lc/LConn1
  Arm_ua/LConn2 -- Series RLC Branch4/LConn1
  Series RLC Branch6/LConn1 -- Arm_uc/LConn2
  Series RLC Branch5/LConn1 -- Series RLC Branch6/RConn1 -- C/RConn1
  Series RLC Branch2/LConn1 -- B/RConn1 -- Series RLC Branch3/RConn1
  Arm_ub/LConn2 -- Series RLC Branch3/LConn1
  Series RLC Branch2/RConn1 -- Arm_lb/LConn1
  Series RLC Branch1/LConn1 -- Series RLC Branch4/RConn1 -- A/RConn1
  Arm_la/LConn2 -- -/RConn1 -- Arm_lc/LConn2 -- Arm_lb/LConn2
  Series RLC Branch1/RConn1 -- Arm_la/LConn1
  Arm_ua/LConn1 -- +/RConn1 -- Arm_uc/LConn1 -- Arm_ub/LConn1

== system GFL_Lib/GFM_VC MMC/Bridge_Model/Modulation Index Generation ==
  vmu_ref : Inport
  vml_ref : Inport  Port=2
  "1 -> Activer filtre notch 0 -> Désactiver filtre notch2" : Constant  Value=Udcn
  Bus Creator : BusCreator  Inputs=6
  Constant : Constant  Value=MMC_Control_Type
  Constant1 : Constant  Value=MMC_Control_Type
  Demux : Demux  Outputs=3
  Demux1 : Demux  Outputs=3
  Demux2 : Demux  Outputs=[3 3]
  Divide1 : Product  Inputs=/*
  Divide4 : Product  Inputs=*/
  Multiport Switch : MultiPortSwitch  Inputs=2
  Multiport Switch1 : MultiPortSwitch  Inputs=2
  Selector : Selector  InputPortWidth=12  IndexOptions=Index vector (dialog)  Indices=[1 2 3 4 5 6]  OutputSizes=1
  m limiter low : Saturate  UpperLimit=1  LowerLimit=0
  m limiter up : Saturate  UpperLimit=1  LowerLimit=0
  mul : Outport
  wires:
  Constant1/1 -> Multiport Switch1/1
  Constant/1 -> Multiport Switch/1
  Demux/3 -> Bus Creator/3  "muc"
  vmu_ref/1 -> Divide1/2
  Multiport Switch/1 -> Divide1/1
  Bus Creator/1 -> mul/1
  Demux1/1 -> Bus Creator/4  "mla"
  Demux1/2 -> Bus Creator/5  "mlb"
  Divide4/1 -> m limiter low/1
  Demux1/3 -> Bus Creator/6  "mlc"
  Multiport Switch1/1 -> Divide4/2
  Demux/2 -> Bus Creator/2  "mub"
  vml_ref/1 -> Divide4/1
  Demux/1 -> Bus Creator/1  "mua"
  m limiter up/1 -> Demux/1
  Divide1/1 -> m limiter up/1
  m limiter low/1 -> Demux1/1
  "1 -> Activer filtre notch 0 -> Désactiver filtre notch2"/1 -> Multiport Switch/2, Multiport Switch1/2
  Selector/1 -> Demux2/1
  [m_mmc] -> Selector/1
  Demux2/1 -> Multiport Switch/3
  Demux2/2 -> Multiport Switch1/3

== system GFL_Lib/GFM_VC MMC/Control loops/ pu P//Q computation ==
  v_abc_pu : Inport  PortDimensions=3
  i_abc_pu : Inport  Port=2  PortDimensions=3
  Demux : Demux  Outputs=3
      settings: DisplayOption=none
  Mux : Mux  Inputs=3
  Product1 : Product  InputSameDT=on  SaturateOnIntegerOverflow=on  OutDataTypeStr=Inherit: Same as first input
  Product3 : Product  InputSameDT=on  SaturateOnIntegerOverflow=on  OutDataTypeStr=Inherit: Same as first input
  Sum : Sum  Inputs=+-  InputSameDT=on  SaturateOnIntegerOverflow=on  OutDataTypeStr=Inherit: Same as first input
  Sum1 : Sum  Inputs=1  InputSameDT=on  SaturateOnIntegerOverflow=on  OutDataTypeStr=Inherit: Same as first input
  Sum4 : Sum  Inputs=1  InputSameDT=on  SaturateOnIntegerOverflow=on  OutDataTypeStr=Inherit: Same as first input
  Sum5 : Sum  Inputs=+-  InputSameDT=on  SaturateOnIntegerOverflow=on  OutDataTypeStr=Inherit: Same as first input
  Sum6 : Sum  Inputs=+-  InputSameDT=on  SaturateOnIntegerOverflow=on  OutDataTypeStr=Inherit: Same as first input
  pu->V : Gain  Gain=1/sqrt(3)  SaturateOnIntegerOverflow=on  OutDataTypeStr=Inherit: Same as input  ParamDataTypeStr=Inherit: Same as input
  pu->V1 : Gain  Gain=1/3  SaturateOnIntegerOverflow=on  OutDataTypeStr=Inherit: Same as input  ParamDataTypeStr=Inherit: Same as input
  pu->V2 : Gain  Gain=1/3  SaturateOnIntegerOverflow=on  OutDataTypeStr=Inherit: Same as input  ParamDataTypeStr=Inherit: Same as input
  P : Outport  VectorParamsAs1DForOutWhenUnconnected=off
  Q : Outport  Port=2  VectorParamsAs1DForOutWhenUnconnected=off
  wires:
  pu->V2/1 -> Q/1
  pu->V1/1 -> P/1
  Sum1/1 -> pu->V/1
  Product3/1 -> Sum1/1
  Product1/1 -> Sum4/1
  v_abc_pu/1 -> Product1/1, Demux/1
  i_abc_pu/1 -> Product1/2, Product3/2
  Sum4/1 -> pu->V1/1
  Demux/1 -> Sum/1, Sum6/2
  Demux/2 -> Sum/2, Sum5/1
  Demux/3 -> Sum5/2, Sum6/1
  Sum/1 -> Mux/3
  Sum5/1 -> Mux/1
  Sum6/1 -> Mux/2
  Mux/1 -> Product3/1
  pu->V/1 -> pu->V2/1  "Q"

== system GFL_Lib/GFM_VC MMC/Control loops/CCSC_dq ==
  Theta : Inport
  Idiff_abc : Inport  Port=2
  Add10 : Sum  Inputs=+-
  Add7 : Sum
  Add8 : Sum
  Add9 : Sum
  Constant : Constant  Value=1/2
  Constant3 : Constant  Value=0
  Constant4 : Constant  Value=0
  Demux : Demux  Outputs=2
  Gain20 : Gain  Gain=-2
  Gain21 : Gain  Gain=Diff_CC_kp
  Gain22 : Gain  Gain=Diff_CC_ki
  Gain23 : Gain  Gain=Diff_CC_kp
  Gain24 : Gain  Gain=Diff_CC_ki
  Gain25 : Gain  Gain=Larm_pu
  Gain26 : Gain  Gain=Larm_pu
  Gain6 : Gain  Gain=1/sqrt(2)
  Integrator1 : Integrator  InitialConditionSource=external
  Integrator3 : Integrator  InitialConditionSource=external
  Mux : Mux  Inputs=2
  Mux4 : Mux  Inputs=2
  Sum : Sum  Inputs=+-
  Sum1 : Sum  Inputs=|+-
  Sum17 : Sum  Inputs=|+-
  Sum18 : Sum  Inputs=-+|
  Sum2 : Sum  Inputs=--|
  Trigonometric Function : Trigonometry  Operator=cos
  Trigonometric Function1 : Trigonometry
  abc2dq0_norm : Control_Lib/abc2dq0_norm  referenceAxisMode=Reference axis at 90 degrees behind phase_a  baseUpdateGain=1/sqrt(3)
      settings: SourceProductName=VSC4SPS
  dq02abc_norm : Control_Lib/dq02abc_norm  referenceAxisMode=Reference axis at 90 degrees behind phase_a  baseUpdateGain=sqrt(3)
      settings: SourceProductName=VSC4SPS
  vdiff_ref : Outport
  wires:
  Sum2/1 -> Integrator3/2
  Sum1/1 -> Integrator1/2
  Constant/1 -> Sum/1
  Sum/1 -> vdiff_ref/1
  Mux4/1 -> dq02abc_norm/1
  abc2dq0_norm/2 -> Demux/1
  Trigonometric Function1/1 -> Mux/2
  Gain20/1 -> Trigonometric Function/1, Trigonometric Function1/1
  Trigonometric Function/1 -> Mux/1
  Gain6/1 -> abc2dq0_norm/1
  dq02abc_norm/2 -> Sum/2
  Gain26/1 -> Add10/2, Sum1/1
  Integrator1/1 -> Add7/1
  Demux/1 -> Sum17/2, Gain25/1
  Gain25/1 -> Add9/2, Sum2/2
  Gain22/1 -> Integrator1/1
  Mux/1 -> abc2dq0_norm/2, dq02abc_norm/3
  Integrator3/1 -> Add8/1
  Add10/1 -> Mux4/1
  Constant4/1 -> Sum18/2
  Sum18/1 -> Gain24/1, Gain23/1
  Add9/1 -> Mux4/2
  Gain23/1 -> Add8/2, Sum2/1
  Gain21/1 -> Add7/2, Sum1/2
  Sum17/1 -> Gain21/1, Gain22/1
  Idiff_abc/1 -> Gain6/1
  Add8/1 -> Add9/1
  Gain24/1 -> Integrator3/1
  Add7/1 -> Add10/1
  Demux/2 -> Gain26/1, Sum18/1
  Constant3/1 -> Sum17/1
  Theta/1 -> Gain20/1

== system GFL_Lib/GFM_VC MMC/Control loops/Current Limitation ==
  note: Current limitation
  Vm_dq* : Inport
  Ig_dq : Inport  Port=2
  vg_dq : Inport  Port=3
  Constant : Constant  Value=I_max_pu
  Current control : Subsystem
  Demux : Demux  Outputs=2
  Demux2 : Demux  Outputs=2
  Inverse Current control : Subsystem
  Mux : Mux  Inputs=2
  Product{,1..3} (4 alike) : Product
  Saturation Dynamic : simulink/Discontinuities/Saturation Dynamic  OutMin=[]  OutMax=[]  OutDataTypeStr=Inherit: Same as second input  OutDataType=fixdt(1, 16)  OutScaling=2^-10  DoSatur=off
  Sqrt : Sqrt  SaturateOnIntegerOverflow=on
  Sum : Sum
  Trigonometric Function : Trigonometry  Operator=atan2  NumberOfIterations=5  OutputSignalType=real
  Trigonometric Function1 : Trigonometry  Operator=cos
  Trigonometric Function2 : Trigonometry
  w_set1 : Constant
  w_set2 : Constant
  w_set3 : Constant  Value=0
  Vm_dq_sat : Outport  VectorParamsAs1DForOutWhenUnconnected=off
  wires:
  w_set3/1 -> Saturation Dynamic/3
  Constant/1 -> Saturation Dynamic/1
  Mux/1 -> Current control/1(Ig_dq0*)
  Product/1 -> Mux/1
  Demux/1 -> Product1/1, Product1/2
  Demux/2 -> Product2/1, Product2/2
  Trigonometric Function2/1 -> Product3/2
  Product2/1 -> Sum/2
  Trigonometric Function1/1 -> Product/2
  Demux2/1 -> Trigonometric Function/2
  Trigonometric Function/1 -> Trigonometric Function2/1, Trigonometric Function1/1
  Saturation Dynamic/1 -> Product/1, Product3/1
  Product1/1 -> Sum/1
  Sqrt/1 -> Saturation Dynamic/2
  Demux2/2 -> Trigonometric Function/1
  Inverse Current control/1(Is_dq*) -> Demux2/1, Demux/1
  Sum/1 -> Sqrt/1
  Product3/1 -> Mux/2
  Ig_dq/1 -> Inverse Current control/2(Ig_dq), Current control/2(Ig_dq0)
  w_set1/1 -> Inverse Current control/4(w)
  w_set2/1 -> Current control/4(w)
  vg_dq/1 -> Current control/3(vg_dq0), Inverse Current control/3(vg_dq)
  Vm_dq*/1 -> Inverse Current control/1(Vm_dq*)
  Current control/1(vm) -> Vm_dq_sat/1

== system GFL_Lib/GFM_VC MMC/Control loops/DC part: stored energy control + differential current control ==
  Wtot_ref_pu : Inport
  theta : Inport  Port=2
  vctot_up_pu : Inport  Port=3
  vctot_low_pu : Inport  Port=4
  Vdc_pu : Inport  Port=5
  pac_pu : Inport  Port=6
  idff_pu : Inport  Port=7
  Constant : Constant  Value=[0 0 0]  SampleTime=-1
  Control Wdiff : Subsystem
  "Control Wtot " : Subsystem
  Differential_current_control : Subsystem
  Sum5 : Sum
  Wdiff computation : Subsystem
  Wtot computation : Subsystem
  vdiff_pu_ref : Outport  PortDimensions=3
  wires:
  Constant/1 -> Control Wdiff/2(Wdiff_ref pu)
  Control Wdiff/1(Idiff ref pu) -> Sum5/2
  Differential_current_control/1(Vprediff_ref_pu) -> vdiff_pu_ref/1
  Vdc_pu/1 -> "Control Wtot "/4(Vdc_pu), Differential_current_control/1(vdc_pu)
  Wtot_ref_pu/1 -> "Control Wtot "/2(Wtot ref pu)
  "Control Wtot "/1(Idiff ref pu) -> Sum5/1
  idff_pu/1 -> Differential_current_control/2(idiff_pu)
  Sum5/1 -> Differential_current_control/3(idiff_ref_pu)
  vctot_up_pu/1 -> Wdiff computation/1(vctot u_pu), Wtot computation/1(vctot u_pu)
  vctot_low_pu/1 -> Wdiff computation/2(vctot l_pu), Wtot computation/2(vctot l_pu)
  Wdiff computation/1(Wdiff) -> Control Wdiff/1(Wdiff pu)
  Wtot computation/1(Wtot) -> "Control Wtot "/1(Wtot_pu)
  theta/1 -> Control Wdiff/3(theta)
  pac_pu/1 -> "Control Wtot "/3(p_ac_pu)

== system GFL_Lib/GFM_VC MMC/Control loops/TVI ==
  note: VI triggering and threshold computation
  note: VI
  i_VI_dq : Inport
  Demux1 : Demux  Outputs=2
      settings: DisplayOption=none
  Gain5 : Gain  Gain=DX_DR
  Gain6 : Gain  Gain=Kp_Rvi_pu
  Gain9 : Gain  Gain=DX_DR
  I_thresh : Constant  Value=I_Max_TVI_pu
  Mux2 : Mux  Inputs=2
  Saturation : Saturate  UpperLimit=inf  LowerLimit=0
  Sum1 : Sum  Inputs=-+|
  Sum7 : Sum  Inputs=|+-
  Sum8 : Sum  Inputs=++|
  dq to phasor : Subsystem
  product{,1..3} (4 alike) : Product  InputSameDT=on  RndMeth=Zero  SaturateOnIntegerOverflow=on  OutDataTypeStr=Inherit: Same as first input
  I_rms : Outport  VectorParamsAs1DForOutWhenUnconnected=off
  Delta_E_dq : Outport  Port=2  VectorParamsAs1DForOutWhenUnconnected=off
  wires:
  Sum1/1 -> Saturation/1
  dq to phasor/1(rms) -> Sum1/2, I_rms/1  "I_rms"
  Saturation/1 -> Gain6/1
  I_thresh/1 -> Sum1/1
  Mux2/1 -> Delta_E_dq/1
  Gain6/1 -> product3/2, product/1, product1/2, product2/2
  product3/1 -> Gain5/1
  product/1 -> Gain9/1
  Demux1/1 -> product1/1, product/2  "igd"
  Demux1/2 -> product2/1, product3/1  "igq"
  product1/1 -> Sum7/1
  Gain5/1 -> Sum7/2
  Gain9/1 -> Sum8/1
  product2/1 -> Sum8/2
  Sum7/1 -> Mux2/1
  Sum8/1 -> Mux2/2
  i_VI_dq/1 -> dq to phasor/1(dq_mes), Demux1/1

== system GFL_Lib/GFM_VC MMC/Control loops/Transient Damping Resistance ==
  ig_dq : Inport
  Filter w_LF : Subsystem
      mask Display: disp('\omega_{LF} / (s + \omega_{LF})','texmode','on')
  Sum5 : Sum  Inputs=|+-
  nq1 : Gain  Gain=Rv
  "Delta_E_dq " : Outport  VectorParamsAs1DForOutWhenUnconnected=off
  wires:
  nq1/1 -> Filter w_LF/1(e), Sum5/2
  Filter w_LF/1(s) -> Sum5/1
  Sum5/1 -> "Delta_E_dq "/1
  ig_dq/1 -> nq1/1

== system GFL_Lib/GFM_VC MMC/Control loops/Vctot_bus_creator ==
  In1 : Inport
  In2 : Inport  Port=2
  Bus Creator1 : BusCreator  Inputs=2
  Bus Creator2 : BusCreator  Inputs=2
  Bus Creator3 : BusCreator  Inputs=2
  Gain : Gain  Gain=Vdcb
  Gain1 : Gain  Gain=Vdcb
  Out1 : Outport
  wires:
  Bus Creator3/1 -> Out1/1
  Gain1/1 -> Bus Creator2/2  "abc"
  Bus Creator2/1 -> Bus Creator3/2  "l"
  In2/1 -> Bus Creator2/1, Gain1/1  "abc_pu"
  In1/1 -> Gain/1, Bus Creator1/1  "abc_pu"
  Bus Creator1/1 -> Bus Creator3/1  "u"
  Gain/1 -> Bus Creator1/2  "abc"

== system GFL_Lib/Mean Model 2-Level L-filter with DC Link/Control loops/ pu P//Q computation ==
  v_abc_pu : Inport  PortDimensions=3
  i_abc_pu : Inport  Port=2  PortDimensions=3
  Demux : Demux  Outputs=3
      settings: DisplayOption=none
  Mux : Mux  Inputs=3
  Product1 : Product  InputSameDT=on  SaturateOnIntegerOverflow=on  OutDataTypeStr=Inherit: Same as first input
  Product3 : Product  InputSameDT=on  SaturateOnIntegerOverflow=on  OutDataTypeStr=Inherit: Same as first input
  Sum : Sum  Inputs=+-  InputSameDT=on  SaturateOnIntegerOverflow=on  OutDataTypeStr=Inherit: Same as first input
  Sum1 : Sum  Inputs=1  InputSameDT=on  SaturateOnIntegerOverflow=on  OutDataTypeStr=Inherit: Same as first input
  Sum4 : Sum  Inputs=1  InputSameDT=on  SaturateOnIntegerOverflow=on  OutDataTypeStr=Inherit: Same as first input
  Sum5 : Sum  Inputs=+-  InputSameDT=on  SaturateOnIntegerOverflow=on  OutDataTypeStr=Inherit: Same as first input
  Sum6 : Sum  Inputs=+-  InputSameDT=on  SaturateOnIntegerOverflow=on  OutDataTypeStr=Inherit: Same as first input
  pu->V : Gain  Gain=1/sqrt(3)  SaturateOnIntegerOverflow=on  OutDataTypeStr=Inherit: Same as input  ParamDataTypeStr=Inherit: Same as input
  pu->V1 : Gain  Gain=1/3  SaturateOnIntegerOverflow=on  OutDataTypeStr=Inherit: Same as input  ParamDataTypeStr=Inherit: Same as input
  pu->V2 : Gain  Gain=1/3  SaturateOnIntegerOverflow=on  OutDataTypeStr=Inherit: Same as input  ParamDataTypeStr=Inherit: Same as input
  P : Outport  VectorParamsAs1DForOutWhenUnconnected=off
  Q : Outport  Port=2  VectorParamsAs1DForOutWhenUnconnected=off
  wires:
  pu->V/1 -> pu->V2/1  "Q"
  Mux/1 -> Product3/1
  Sum6/1 -> Mux/2
  Sum5/1 -> Mux/1
  Sum/1 -> Mux/3
  Demux/3 -> Sum6/1, Sum5/2
  Demux/2 -> Sum5/1, Sum/2
  Demux/1 -> Sum6/2, Sum/1
  Sum4/1 -> pu->V1/1
  i_abc_pu/1 -> Product3/2, Product1/2
  v_abc_pu/1 -> Demux/1, Product1/1
  Product1/1 -> Sum4/1
  Product3/1 -> Sum1/1
  Sum1/1 -> pu->V/1
  pu->V1/1 -> P/1
  pu->V2/1 -> Q/1

== system GFL_Lib/Mean Model 2-Level L-filter with DC Link/Control loops/Inner Current Control ==
  ig_dq_ref : Inport
  ig_dq : Inport  Port=2
  w_PLL : Inport  Port=3
  vg_dq : Inport  Port=4
  ig_dq_max : Inport  Port=5
  Current PI control : Subsystem
  vm_dq : Outport  VectorParamsAs1DForOutWhenUnconnected=off
  wires:
  w_PLL/1 -> Current PI control/4(w)  "w"
  vg_dq/1 -> Current PI control/2(Eg_dqfr)  "Eg_dq"
  ig_dq_ref/1 -> Current PI control/3(Is_dq_ref)
  Current PI control/1(vm_dq_ref) -> vm_dq/1  "vm_dq"
  ig_dq/1 -> Current PI control/1(Is_dq)  "Is_dq"
  ig_dq_max/1 -> Current PI control/5(Idq_ref_max)

== system GFL_Lib/Mean Model 2-Level L-filter with DC Link/Control loops/LPF ==
  In1 : Inport
  Add : Sum  Inputs=+-
  Gain : Gain  Gain=w_LPF
  Integrator : Integrator  InitialCondition=P0
  Out1 : Outport
  wires:
  In1/1 -> Add/1
  Integrator/1 -> Add/2, Out1/1
  Gain/1 -> Integrator/1
  Add/1 -> Gain/1

== system GFL_Lib/Mean Model 2-Level L-filter with DC Link/Control loops/LPF1 ==
  In1 : Inport
  Add : Sum  Inputs=+-
  Gain : Gain  Gain=w_LPF
  Integrator : Integrator  InitialCondition=V0
  Out1 : Outport
  wires:
  In1/1 -> Add/1
  Integrator/1 -> Add/2, Out1/1
  Gain/1 -> Integrator/1
  Add/1 -> Gain/1

== system GFL_Lib/Mean Model 2-Level L-filter with DC Link/Control loops/LPF2 ==
  In1 : Inport
  Add : Sum  Inputs=+-
  Gain : Gain  Gain=w_LPF
  Integrator : Integrator  InitialCondition=Q0
  Out1 : Outport
  wires:
  In1/1 -> Add/1
  Integrator/1 -> Add/2, Out1/1
  Gain/1 -> Integrator/1
  Add/1 -> Gain/1

== system GFL_Lib/Mean Model 2-Level L-filter with DC Link/Control loops/LPF3 ==
  In1 : Inport
  Add : Sum  Inputs=+-
  Gain : Gain  Gain=2*pi*50
  Integrator : Integrator  InitialCondition=V0
  Out1 : Outport
  wires:
  In1/1 -> Add/1
  Integrator/1 -> Add/2, Out1/1
  Gain/1 -> Integrator/1
  Add/1 -> Gain/1

== system GFL_Lib/Mean Model 2-Level L-filter with DC Link/Control loops/RMS derivation ==
  dq : Inport
  Demux : Demux  Outputs=2
  Sqrt : Sqrt  SaturateOnIntegerOverflow=on
  Square : Math  Operator=square  SaturateOnIntegerOverflow=on
  Square1 : Math  Operator=square  SaturateOnIntegerOverflow=on
  Sum : Sum
  rms : Outport
  wires:
  dq/1 -> Demux/1
  Demux/2 -> Square1/1
  Square/1 -> Sum/1
  Demux/1 -> Square/1
  Sqrt/1 -> rms/1
  Sum/1 -> Sqrt/1
  Square1/1 -> Sum/2

== system GFL_Lib/Mean Model 2-Level L-filter with DC Link/Control loops/norm1 ==
  In1 : Inport
  Add : Sum
  Demux : Demux  Outputs=2
  Sqrt : Sqrt  SaturateOnIntegerOverflow=on
  Square : Math  Operator=square  SaturateOnIntegerOverflow=on
  Square1 : Math  Operator=square  SaturateOnIntegerOverflow=on
  Out1 : Outport
  wires:
  In1/1 -> Demux/1
  Square1/1 -> Add/2
  Square/1 -> Add/1
  Demux/1 -> Square/1
  Demux/2 -> Square1/1
  Add/1 -> Sqrt/1
  Sqrt/1 -> Out1/1

== system GFL_Lib/Mean Model 2-Level L-filter with DC Link/Control loops/norm2 ==
  In1 : Inport
  Add : Sum
  Demux : Demux  Outputs=2
  Sqrt : Sqrt  SaturateOnIntegerOverflow=on
  Square : Math  Operator=square  SaturateOnIntegerOverflow=on
  Square1 : Math  Operator=square  SaturateOnIntegerOverflow=on
  Out1 : Outport
  wires:
  In1/1 -> Demux/1
  Square1/1 -> Add/2
  Square/1 -> Add/1
  Demux/1 -> Square/1
  Demux/2 -> Square1/1
  Add/1 -> Sqrt/1
  Sqrt/1 -> Out1/1

== system GFL_Lib/Mean Model 2-Level L-filter_old/Control loops/ pu P//Q computation ==
  v_abc_pu : Inport  PortDimensions=3
  i_abc_pu : Inport  Port=2  PortDimensions=3
  Demux : Demux  Outputs=3
      settings: DisplayOption=none
  Mux : Mux  Inputs=3
  Product1 : Product  InputSameDT=on  SaturateOnIntegerOverflow=on  OutDataTypeStr=Inherit: Same as first input
  Product3 : Product  InputSameDT=on  SaturateOnIntegerOverflow=on  OutDataTypeStr=Inherit: Same as first input
  Sum : Sum  Inputs=+-  InputSameDT=on  SaturateOnIntegerOverflow=on  OutDataTypeStr=Inherit: Same as first input
  Sum1 : Sum  Inputs=1  InputSameDT=on  SaturateOnIntegerOverflow=on  OutDataTypeStr=Inherit: Same as first input
  Sum4 : Sum  Inputs=1  InputSameDT=on  SaturateOnIntegerOverflow=on  OutDataTypeStr=Inherit: Same as first input
  Sum5 : Sum  Inputs=+-  InputSameDT=on  SaturateOnIntegerOverflow=on  OutDataTypeStr=Inherit: Same as first input
  Sum6 : Sum  Inputs=+-  InputSameDT=on  SaturateOnIntegerOverflow=on  OutDataTypeStr=Inherit: Same as first input
  pu->V : Gain  Gain=1/sqrt(3)  SaturateOnIntegerOverflow=on  OutDataTypeStr=Inherit: Same as input  ParamDataTypeStr=Inherit: Same as input
  pu->V1 : Gain  Gain=1/3  SaturateOnIntegerOverflow=on  OutDataTypeStr=Inherit: Same as input  ParamDataTypeStr=Inherit: Same as input
  pu->V2 : Gain  Gain=1/3  SaturateOnIntegerOverflow=on  OutDataTypeStr=Inherit: Same as input  ParamDataTypeStr=Inherit: Same as input
  P : Outport  VectorParamsAs1DForOutWhenUnconnected=off
  Q : Outport  Port=2  VectorParamsAs1DForOutWhenUnconnected=off
  wires:
  pu->V/1 -> pu->V2/1  "Q"
  Mux/1 -> Product3/1
  Sum6/1 -> Mux/2
  Sum5/1 -> Mux/1
  Sum/1 -> Mux/3
  Demux/3 -> Sum6/1, Sum5/2
  Demux/2 -> Sum5/1, Sum/2
  Demux/1 -> Sum6/2, Sum/1
  Sum4/1 -> pu->V1/1
  i_abc_pu/1 -> Product3/2, Product1/2
  v_abc_pu/1 -> Demux/1, Product1/1
  Product1/1 -> Sum4/1
  Product3/1 -> Sum1/1
  Sum1/1 -> pu->V/1
  pu->V1/1 -> P/1
  pu->V2/1 -> Q/1

== system GFL_Lib/Mean Model 2-Level L-filter_old/Control loops/Inner Current Control ==
  ig_dq_ref : Inport
  ig_dq : Inport  Port=2
  w_PLL : Inport  Port=3
  vg_dq : Inport  Port=4
  ig_dq_max : Inport  Port=5
  Current PI control : Subsystem
  vm_dq : Outport  VectorParamsAs1DForOutWhenUnconnected=off
  wires:
  w_PLL/1 -> Current PI control/4(w)  "w"
  vg_dq/1 -> Current PI control/2(Eg_dqfr)  "Eg_dq"
  ig_dq_ref/1 -> Current PI control/3(Is_dq_ref)
  Current PI control/1(vm_dq_ref) -> vm_dq/1  "vm_dq"
  ig_dq/1 -> Current PI control/1(Is_dq)  "Is_dq"
  ig_dq_max/1 -> Current PI control/5(Idq_ref_max)

== system GFL_Lib/Mean Model 2-Level L-filter_old/Control loops/LPF ==
  In1 : Inport
  Add : Sum  Inputs=+-
  Gain : Gain  Gain=w_LPF
  Integrator : Integrator  InitialCondition=P0
  Out1 : Outport
  wires:
  In1/1 -> Add/1
  Integrator/1 -> Add/2, Out1/1
  Gain/1 -> Integrator/1
  Add/1 -> Gain/1

== system GFL_Lib/Mean Model 2-Level L-filter_old/Control loops/LPF1 ==
  In1 : Inport
  Add : Sum  Inputs=+-
  Gain : Gain  Gain=w_LPF
  Integrator : Integrator  InitialCondition=V0
  Out1 : Outport
  wires:
  In1/1 -> Add/1
  Integrator/1 -> Add/2, Out1/1
  Gain/1 -> Integrator/1
  Add/1 -> Gain/1

== system GFL_Lib/Mean Model 2-Level L-filter_old/Control loops/LPF2 ==
  In1 : Inport
  Add : Sum  Inputs=+-
  Gain : Gain  Gain=w_LPF
  Integrator : Integrator  InitialCondition=Q0
  Out1 : Outport
  wires:
  In1/1 -> Add/1
  Integrator/1 -> Add/2, Out1/1
  Gain/1 -> Integrator/1
  Add/1 -> Gain/1
